simulink model "TSR_Scenario_005_cs"  (R2014b)
settings: Solver=ode5  SolverMode=SingleTasking  StartTime=0.0  StopTime=inf  FixedStep=1/100  RelTol=1e-3
PreLoadFcn:
  | mbxruntime.callbacks.PreLoadFcn(bdroot);
  | check_NUTS_defined;
  | 
  | assignin('base',['model_closed_' bdroot],false);
  | 
  | addpath('../includes_TSR/includes_TSR');
  | 
  | switch version('-release')
  | case {'2010a', '2010b', '2011a'}
  | addpath('../includes_TSR/ML2010b');
  | otherwise
  | addpath('../includes_TSR/ML2011b');
  | end
PostLoadFcn:
  | mbxruntime.callbacks.PostLoadFcn(bdroot);
InitFcn:
  | mbxruntime.callbacks.InitFcn(bdroot);
StartFcn:
  | mbxruntime.callbacks.StartFcn(bdroot);
StopFcn:
  | mbxruntime.callbacks.StopFcn(bdroot);
model workspace: external: MAT-File .\TSR_Scenario_005_cs_hws.mat (data not in the file)
undefined symbols (not defined in the file or in its folder): InitImageOutputDir, mbxruntime, OrientationPitch, OrientationRoll, PositionX, PositionY, PositionZ, tabledata, warningInitialVelocity, x0
undefined symbols (not defined in the file): SteeringColumn, SteeringWheel, TSR_Scenario_005_cs_00431f954bf6ed0a, TSR_Scenario_005_cs_02a6645fe307ce96, TSR_Scenario_005_cs_0e0d17e780cba748, TSR_Scenario_005_cs_0f94700004e304be, TSR_Scenario_005_cs_13e63084604f23c5, TSR_Scenario_005_cs_18da76569b226b1d, TSR_Scenario_005_cs_19a09eb0dceaf389, TSR_Scenario_005_cs_1d6b1ecf339da803, TSR_Scenario_005_cs_219485daa5a5d171, TSR_Scenario_005_cs_221c03cfb0670d1a, TSR_Scenario_005_cs_22611db63f83df91, TSR_Scenario_005_cs_24324341e1f0fdeb, TSR_Scenario_005_cs_248b5be6aaeb4a32, TSR_Scenario_005_cs_26d69342f02903e6, TSR_Scenario_005_cs_28d4639b4eb6a924, TSR_Scenario_005_cs_2a50646ef6121283, TSR_Scenario_005_cs_2addef8764f78195, TSR_Scenario_005_cs_2c78bb6e92f1c73d, TSR_Scenario_005_cs_330b013c7926b8c0, TSR_Scenario_005_cs_33ac55a3a4bfafc5, TSR_Scenario_005_cs_33d6442482a921b6, TSR_Scenario_005_cs_36fcc85960c1dc31, TSR_Scenario_005_cs_38acb22310967a91, TSR_Scenario_005_cs_3e8855054a9c05f5, TSR_Scenario_005_cs_43d01b44652f0f38, TSR_Scenario_005_cs_43d19ecb630bd754, TSR_Scenario_005_cs_4487c76a87b8c5f1, TSR_Scenario_005_cs_44ceee846c318dfb, TSR_Scenario_005_cs_450a3683cbfdd730, TSR_Scenario_005_cs_464618e49e37493a, TSR_Scenario_005_cs_4880b38df4698ab1, TSR_Scenario_005_cs_4a2b3c7d0abca22e, TSR_Scenario_005_cs_4bd204b8239d5406, TSR_Scenario_005_cs_4de8d67ffbf74a19, TSR_Scenario_005_cs_4f6170ee339e194e, TSR_Scenario_005_cs_50430c8166448bfc, TSR_Scenario_005_cs_53c8f6734eaacbd2, TSR_Scenario_005_cs_543db9a2ff458ebe, TSR_Scenario_005_cs_57976f30ab2edad5, TSR_Scenario_005_cs_5922fccf31372278, TSR_Scenario_005_cs_5a258c940bbe826b, TSR_Scenario_005_cs_6087cc283675db35, TSR_Scenario_005_cs_6246b869963d4acb, TSR_Scenario_005_cs_6352b9f9b72630f9, TSR_Scenario_005_cs_6559b64eceddc3ca, TSR_Scenario_005_cs_6832a8ea8fa66aa4, TSR_Scenario_005_cs_696d53dba69844e5, TSR_Scenario_005_cs_6cabbb37c4ac2dd1, TSR_Scenario_005_cs_6d528aa494c8a952, TSR_Scenario_005_cs_6d945b49f7234fd2, TSR_Scenario_005_cs_6e2ebc771acb2455, TSR_Scenario_005_cs_7897f864ad990cf0, TSR_Scenario_005_cs_7978c65fd141f076, TSR_Scenario_005_cs_7a9ba94120bbe2c7, TSR_Scenario_005_cs_7b108592703c2dc5, TSR_Scenario_005_cs_7cd2f5b09394b811, TSR_Scenario_005_cs_7e1904d085d8f37f, TSR_Scenario_005_cs_7e555208507e0618 ... (+95)
libraries: simulink_extras x59, PreScanSimulinkLibrary x43, simulink x29
(part 6 of 24)

== system TSR_Scenario_005_cs/Lightpost_27 ==
  note: Texture Resources for Light
      |
      | ID: resource name
      | 1: LightMap\HeadLight LB and HB.png: HeadLight LB and HB
      | 2: LightMap\HeadLight LB.png: HeadLight LB
      | 3: LightMap\GeneralLight.png: GeneralLight
      | 4: LightMap\BrakeLight.png: BrakeLight
      | 5: LightMap\RearLight.png: RearLight
      | 6: LightMap\HeadLight HB.png: HeadLight HB
  Light_Col : Constant  Tag=VisuLightConst  Value=[255 210 89]
  Light_ID : Constant  Tag=VisuLightConst  Value=[0]
  Light_Mux : Subsystem  Tag=mux/ActiveLight  mask(PreScan User Interface: VisuActiveLight){}
      mask help:
      | The VisuActiveLight block provides a way for detailed animation of Light Sources, such as the indicator, brake, fog and main lights of a vehicle, or a light post.
      |
      | For more information, please click Help.
      settings: DeleteFcn=PreScanBlockDeleteFcn;
      mask Help: eval('openHelp(209)')
  Light_Ori : Constant  Tag=VisuLightConst  Value=[0.000000 -0.000000 0.000000]
  Light_Pos : Constant  Tag=VisuLightConst  Value=[-0.038900 -0.000018 0.870000]
  Light_mscd : Constant  Tag=VisuLightConst  Value=[48.371371]
  Lightpost_27_Light : Outport  Tag=outport/Light  OutDataTypeStr=Bus: PRESCAN_VISULIGHTACTUATOR_DATA  SampleTime=1/100
  wires:
  Light_Mux/1(Lights) -> Lightpost_27_Light/1
  Light_mscd/1 -> Light_Mux/1(MSCD [Cd])
  Light_Pos/1 -> Light_Mux/2(Position (xyz) [m])
  Light_Ori/1 -> Light_Mux/3(Orientation (RPY) [deg])
  Light_Col/1 -> Light_Mux/4(Color [-])
  Light_ID/1 -> Light_Mux/5(TextureResourceID [-])

== system TSR_Scenario_005_cs/Lightpost_27_Light ==
  Lightpost_27_Light : Inport  Tag=inport/Light  OutDataTypeStr=Bus: PRESCAN_VISULIGHTACTUATOR_DATA  SampleTime=1/100  BusOutputAsStruct=on
  Actuator : S-Function  FunctionName=sfun_VisuLightActuator  Parameters=mbxruntime.parameters.convert(UniqueID), mbxruntime.parameters.convert(LightName), mbxruntime.parameters.convert(PivotName), mbxruntime.parameters.convert(TextureResources), mbxruntime.parameters.convert(ColorsObjectName), mbxruntime.parameters.convert(MeshOnColor), mbxruntime.parameters.convert(MeshOffColor),tabledata, TimeStep  EnableBusSupport=off  mask(PreScan Sink Block: VisuActiveLight){UniqueID=638, LightName=Lightpost_27.LightActuator_0_Light_ActiveLight, PivotName=Lightpost_27.Light, TextureResources={ '1' 'LightMap\HeadLight LB and HB.png' '2' 'LightMap\HeadLight LB.png' '3' 'LightMap\GeneralLight.png' '4' 'LightMap\BrakeLight.png' '5' 'LightMap\RearLight.png' '6' 'LightMap\HeadLight HB.png'}, ColorsObjectName=Lightpost_27.Light, MeshOnColor=[224  224  224  255  224  224  224  255  102  102  102  255  510  420  178  255], MeshOffColor=[224  224  224  255  224  224  224  255  102  102  102  255    0    0    0  255], TimeStep=1/100}
      mask prompts: UniqueID "Parent Unique Identifier"; LightName "Light"; PivotName "Pivot"; TextureResources "Texture Resources"; ColorsObjectName "Light Fixture Color Object"; MeshOnColor "Light Fixture On Color"; MeshOffColor "Light Fixture Off Color"; TimeStep "Simulink time step"
      mask help:
      | The VisuActiveLight block provides a way for detailed animation of Light Sources, such as the indicator, brake, fog and main lights of a vehicle, or a light post.
      |
      | For more information, please click Help.
      mask init:
      | [tabledata] = mbxruntime.parameters.table(UniqueID,LightName,PivotName,TextureResources,ColorsObjectName,MeshOnColor,MeshOffColor);
      mask Help: eval('openHelp(209)')
      mask Display: image(imread('HeadLight.png'))
  wires:
  Lightpost_27_Light/1 -> Actuator/1

== system TSR_Scenario_005_cs/Lightpost_2_Light ==
  Lightpost_2_Light : Inport  Tag=inport/Light  OutDataTypeStr=Bus: PRESCAN_VISULIGHTACTUATOR_DATA  SampleTime=1/100  BusOutputAsStruct=on
  Actuator : S-Function  FunctionName=sfun_VisuLightActuator  Parameters=mbxruntime.parameters.convert(UniqueID), mbxruntime.parameters.convert(LightName), mbxruntime.parameters.convert(PivotName), mbxruntime.parameters.convert(TextureResources), mbxruntime.parameters.convert(ColorsObjectName), mbxruntime.parameters.convert(MeshOnColor), mbxruntime.parameters.convert(MeshOffColor),tabledata, TimeStep  EnableBusSupport=off  mask(PreScan Sink Block: VisuActiveLight){UniqueID=148, LightName=Lightpost_2.LightActuator_0_Light_ActiveLight, PivotName=Lightpost_2.Light, TextureResources={ '1' 'LightMap\HeadLight LB and HB.png' '2' 'LightMap\HeadLight LB.png' '3' 'LightMap\GeneralLight.png' '4' 'LightMap\BrakeLight.png' '5' 'LightMap\RearLight.png' '6' 'LightMap\HeadLight HB.png'}, ColorsObjectName=Lightpost_2.Light, MeshOnColor=[224  224  224  255  224  224  224  255  102  102  102  255  510  420  178  255], MeshOffColor=[224  224  224  255  224  224  224  255  102  102  102  255    0    0    0  255], TimeStep=1/100}
      mask prompts: UniqueID "Parent Unique Identifier"; LightName "Light"; PivotName "Pivot"; TextureResources "Texture Resources"; ColorsObjectName "Light Fixture Color Object"; MeshOnColor "Light Fixture On Color"; MeshOffColor "Light Fixture Off Color"; TimeStep "Simulink time step"
      mask help:
      | The VisuActiveLight block provides a way for detailed animation of Light Sources, such as the indicator, brake, fog and main lights of a vehicle, or a light post.
      |
      | For more information, please click Help.
      mask init:
      | [tabledata] = mbxruntime.parameters.table(UniqueID,LightName,PivotName,TextureResources,ColorsObjectName,MeshOnColor,MeshOffColor);
      mask Help: eval('openHelp(209)')
      mask Display: image(imread('HeadLight.png'))
  wires:
  Lightpost_2_Light/1 -> Actuator/1

== system TSR_Scenario_005_cs/Lightpost_3 ==
  note: Texture Resources for Light
      |
      | ID: resource name
      | 1: LightMap\HeadLight LB and HB.png: HeadLight LB and HB
      | 2: LightMap\HeadLight LB.png: HeadLight LB
      | 3: LightMap\GeneralLight.png: GeneralLight
      | 4: LightMap\BrakeLight.png: BrakeLight
      | 5: LightMap\RearLight.png: RearLight
      | 6: LightMap\HeadLight HB.png: HeadLight HB
  Light_Col : Constant  Tag=VisuLightConst  Value=[255 210 89]
  Light_ID : Constant  Tag=VisuLightConst  Value=[0]
  Light_Mux : Subsystem  Tag=mux/ActiveLight  mask(PreScan User Interface: VisuActiveLight){}
      mask help:
      | The VisuActiveLight block provides a way for detailed animation of Light Sources, such as the indicator, brake, fog and main lights of a vehicle, or a light post.
      |
      | For more information, please click Help.
      settings: DeleteFcn=PreScanBlockDeleteFcn;
      mask Help: eval('openHelp(209)')
  Light_Ori : Constant  Tag=VisuLightConst  Value=[0.000000 -0.000000 0.000000]
  Light_Pos : Constant  Tag=VisuLightConst  Value=[-0.038900 -0.000018 0.870000]
  Light_mscd : Constant  Tag=VisuLightConst  Value=[48.371371]
  Lightpost_3_Light : Outport  Tag=outport/Light  OutDataTypeStr=Bus: PRESCAN_VISULIGHTACTUATOR_DATA  SampleTime=1/100
  wires:
  Light_Mux/1(Lights) -> Lightpost_3_Light/1
  Light_mscd/1 -> Light_Mux/1(MSCD [Cd])
  Light_Pos/1 -> Light_Mux/2(Position (xyz) [m])
  Light_Ori/1 -> Light_Mux/3(Orientation (RPY) [deg])
  Light_Col/1 -> Light_Mux/4(Color [-])
  Light_ID/1 -> Light_Mux/5(TextureResourceID [-])

== system TSR_Scenario_005_cs/Lightpost_34 ==
  note: Texture Resources for Light
      |
      | ID: resource name
      | 1: LightMap\HeadLight LB and HB.png: HeadLight LB and HB
      | 2: LightMap\HeadLight LB.png: HeadLight LB
      | 3: LightMap\GeneralLight.png: GeneralLight
      | 4: LightMap\BrakeLight.png: BrakeLight
      | 5: LightMap\RearLight.png: RearLight
      | 6: LightMap\HeadLight HB.png: HeadLight HB
  Light_Col : Constant  Tag=VisuLightConst  Value=[255 210 89]
  Light_ID : Constant  Tag=VisuLightConst  Value=[0]
  Light_Mux : Subsystem  Tag=mux/ActiveLight  mask(PreScan User Interface: VisuActiveLight){}
      mask help:
      | The VisuActiveLight block provides a way for detailed animation of Light Sources, such as the indicator, brake, fog and main lights of a vehicle, or a light post.
      |
      | For more information, please click Help.
      settings: DeleteFcn=PreScanBlockDeleteFcn;
      mask Help: eval('openHelp(209)')
  Light_Ori : Constant  Tag=VisuLightConst  Value=[0.000000 -0.000000 0.000000]
  Light_Pos : Constant  Tag=VisuLightConst  Value=[-0.038900 -0.000018 0.870000]
  Light_mscd : Constant  Tag=VisuLightConst  Value=[48.371371]
  Lightpost_34_Light : Outport  Tag=outport/Light  OutDataTypeStr=Bus: PRESCAN_VISULIGHTACTUATOR_DATA  SampleTime=1/100
  wires:
  Light_Mux/1(Lights) -> Lightpost_34_Light/1
  Light_mscd/1 -> Light_Mux/1(MSCD [Cd])
  Light_Pos/1 -> Light_Mux/2(Position (xyz) [m])
  Light_Ori/1 -> Light_Mux/3(Orientation (RPY) [deg])
  Light_Col/1 -> Light_Mux/4(Color [-])
  Light_ID/1 -> Light_Mux/5(TextureResourceID [-])

== system TSR_Scenario_005_cs/Lightpost_34_Light ==
  Lightpost_34_Light : Inport  Tag=inport/Light  OutDataTypeStr=Bus: PRESCAN_VISULIGHTACTUATOR_DATA  SampleTime=1/100  BusOutputAsStruct=on
  Actuator : S-Function  FunctionName=sfun_VisuLightActuator  Parameters=mbxruntime.parameters.convert(UniqueID), mbxruntime.parameters.convert(LightName), mbxruntime.parameters.convert(PivotName), mbxruntime.parameters.convert(TextureResources), mbxruntime.parameters.convert(ColorsObjectName), mbxruntime.parameters.convert(MeshOnColor), mbxruntime.parameters.convert(MeshOffColor),tabledata, TimeStep  EnableBusSupport=off  mask(PreScan Sink Block: VisuActiveLight){UniqueID=645, LightName=Lightpost_34.LightActuator_0_Light_ActiveLight, PivotName=Lightpost_34.Light, TextureResources={ '1' 'LightMap\HeadLight LB and HB.png' '2' 'LightMap\HeadLight LB.png' '3' 'LightMap\GeneralLight.png' '4' 'LightMap\BrakeLight.png' '5' 'LightMap\RearLight.png' '6' 'LightMap\HeadLight HB.png'}, ColorsObjectName=Lightpost_34.Light, MeshOnColor=[224  224  224  255  224  224  224  255  102  102  102  255  510  420  178  255], MeshOffColor=[224  224  224  255  224  224  224  255  102  102  102  255    0    0    0  255], TimeStep=1/100}
      mask prompts: UniqueID "Parent Unique Identifier"; LightName "Light"; PivotName "Pivot"; TextureResources "Texture Resources"; ColorsObjectName "Light Fixture Color Object"; MeshOnColor "Light Fixture On Color"; MeshOffColor "Light Fixture Off Color"; TimeStep "Simulink time step"
      mask help:
      | The VisuActiveLight block provides a way for detailed animation of Light Sources, such as the indicator, brake, fog and main lights of a vehicle, or a light post.
      |
      | For more information, please click Help.
      mask init:
      | [tabledata] = mbxruntime.parameters.table(UniqueID,LightName,PivotName,TextureResources,ColorsObjectName,MeshOnColor,MeshOffColor);
      mask Help: eval('openHelp(209)')
      mask Display: image(imread('HeadLight.png'))
  wires:
  Lightpost_34_Light/1 -> Actuator/1

== system TSR_Scenario_005_cs/Lightpost_36 ==
  note: Texture Resources for Light
      |
      | ID: resource name
      | 1: LightMap\HeadLight LB and HB.png: HeadLight LB and HB
      | 2: LightMap\HeadLight LB.png: HeadLight LB
      | 3: LightMap\GeneralLight.png: GeneralLight
      | 4: LightMap\BrakeLight.png: BrakeLight
      | 5: LightMap\RearLight.png: RearLight
      | 6: LightMap\HeadLight HB.png: HeadLight HB
  Light_Col : Constant  Tag=VisuLightConst  Value=[255 210 89]
  Light_ID : Constant  Tag=VisuLightConst  Value=[0]
  Light_Mux : Subsystem  Tag=mux/ActiveLight  mask(PreScan User Interface: VisuActiveLight){}
      mask help:
      | The VisuActiveLight block provides a way for detailed animation of Light Sources, such as the indicator, brake, fog and main lights of a vehicle, or a light post.
      |
      | For more information, please click Help.
      settings: DeleteFcn=PreScanBlockDeleteFcn;
      mask Help: eval('openHelp(209)')
  Light_Ori : Constant  Tag=VisuLightConst  Value=[0.000000 -0.000000 0.000000]
  Light_Pos : Constant  Tag=VisuLightConst  Value=[-0.038900 -0.000018 0.870000]
  Light_mscd : Constant  Tag=VisuLightConst  Value=[48.371371]
  Lightpost_36_Light : Outport  Tag=outport/Light  OutDataTypeStr=Bus: PRESCAN_VISULIGHTACTUATOR_DATA  SampleTime=1/100
  wires:
  Light_Mux/1(Lights) -> Lightpost_36_Light/1
  Light_mscd/1 -> Light_Mux/1(MSCD [Cd])
  Light_Pos/1 -> Light_Mux/2(Position (xyz) [m])
  Light_Ori/1 -> Light_Mux/3(Orientation (RPY) [deg])
  Light_Col/1 -> Light_Mux/4(Color [-])
  Light_ID/1 -> Light_Mux/5(TextureResourceID [-])

== system TSR_Scenario_005_cs/Lightpost_36_Light ==
  Lightpost_36_Light : Inport  Tag=inport/Light  OutDataTypeStr=Bus: PRESCAN_VISULIGHTACTUATOR_DATA  SampleTime=1/100  BusOutputAsStruct=on
  Actuator : S-Function  FunctionName=sfun_VisuLightActuator  Parameters=mbxruntime.parameters.convert(UniqueID), mbxruntime.parameters.convert(LightName), mbxruntime.parameters.convert(PivotName), mbxruntime.parameters.convert(TextureResources), mbxruntime.parameters.convert(ColorsObjectName), mbxruntime.parameters.convert(MeshOnColor), mbxruntime.parameters.convert(MeshOffColor),tabledata, TimeStep  EnableBusSupport=off  mask(PreScan Sink Block: VisuActiveLight){UniqueID=647, LightName=Lightpost_36.LightActuator_0_Light_ActiveLight, PivotName=Lightpost_36.Light, TextureResources={ '1' 'LightMap\HeadLight LB and HB.png' '2' 'LightMap\HeadLight LB.png' '3' 'LightMap\GeneralLight.png' '4' 'LightMap\BrakeLight.png' '5' 'LightMap\RearLight.png' '6' 'LightMap\HeadLight HB.png'}, ColorsObjectName=Lightpost_36.Light, MeshOnColor=[224  224  224  255  224  224  224  255  102  102  102  255  510  420  178  255], MeshOffColor=[224  224  224  255  224  224  224  255  102  102  102  255    0    0    0  255], TimeStep=1/100}
      mask prompts: UniqueID "Parent Unique Identifier"; LightName "Light"; PivotName "Pivot"; TextureResources "Texture Resources"; ColorsObjectName "Light Fixture Color Object"; MeshOnColor "Light Fixture On Color"; MeshOffColor "Light Fixture Off Color"; TimeStep "Simulink time step"
      mask help:
      | The VisuActiveLight block provides a way for detailed animation of Light Sources, such as the indicator, brake, fog and main lights of a vehicle, or a light post.
      |
      | For more information, please click Help.
      mask init:
      | [tabledata] = mbxruntime.parameters.table(UniqueID,LightName,PivotName,TextureResources,ColorsObjectName,MeshOnColor,MeshOffColor);
      mask Help: eval('openHelp(209)')
      mask Display: image(imread('HeadLight.png'))
  wires:
  Lightpost_36_Light/1 -> Actuator/1

== system TSR_Scenario_005_cs/Lightpost_38 ==
  note: Texture Resources for Light
      |
      | ID: resource name
      | 1: LightMap\HeadLight LB and HB.png: HeadLight LB and HB
      | 2: LightMap\HeadLight LB.png: HeadLight LB
      | 3: LightMap\GeneralLight.png: GeneralLight
      | 4: LightMap\BrakeLight.png: BrakeLight
      | 5: LightMap\RearLight.png: RearLight
      | 6: LightMap\HeadLight HB.png: HeadLight HB
  Light_Col : Constant  Tag=VisuLightConst  Value=[255 210 89]
  Light_ID : Constant  Tag=VisuLightConst  Value=[0]
  Light_Mux : Subsystem  Tag=mux/ActiveLight  mask(PreScan User Interface: VisuActiveLight){}
      mask help:
      | The VisuActiveLight block provides a way for detailed animation of Light Sources, such as the indicator, brake, fog and main lights of a vehicle, or a light post.
      |
      | For more information, please click Help.
      settings: DeleteFcn=PreScanBlockDeleteFcn;
      mask Help: eval('openHelp(209)')
  Light_Ori : Constant  Tag=VisuLightConst  Value=[0.000000 -0.000000 0.000000]
  Light_Pos : Constant  Tag=VisuLightConst  Value=[-0.038900 -0.000018 0.870000]
  Light_mscd : Constant  Tag=VisuLightConst  Value=[48.371371]
  Lightpost_38_Light : Outport  Tag=outport/Light  OutDataTypeStr=Bus: PRESCAN_VISULIGHTACTUATOR_DATA  SampleTime=1/100
  wires:
  Light_Mux/1(Lights) -> Lightpost_38_Light/1
  Light_mscd/1 -> Light_Mux/1(MSCD [Cd])
  Light_Pos/1 -> Light_Mux/2(Position (xyz) [m])
  Light_Ori/1 -> Light_Mux/3(Orientation (RPY) [deg])
  Light_Col/1 -> Light_Mux/4(Color [-])
  Light_ID/1 -> Light_Mux/5(TextureResourceID [-])

== system TSR_Scenario_005_cs/Lightpost_38_Light ==
  Lightpost_38_Light : Inport  Tag=inport/Light  OutDataTypeStr=Bus: PRESCAN_VISULIGHTACTUATOR_DATA  SampleTime=1/100  BusOutputAsStruct=on
  Actuator : S-Function  FunctionName=sfun_VisuLightActuator  Parameters=mbxruntime.parameters.convert(UniqueID), mbxruntime.parameters.convert(LightName), mbxruntime.parameters.convert(PivotName), mbxruntime.parameters.convert(TextureResources), mbxruntime.parameters.convert(ColorsObjectName), mbxruntime.parameters.convert(MeshOnColor), mbxruntime.parameters.convert(MeshOffColor),tabledata, TimeStep  EnableBusSupport=off  mask(PreScan Sink Block: VisuActiveLight){UniqueID=649, LightName=Lightpost_38.LightActuator_0_Light_ActiveLight, PivotName=Lightpost_38.Light, TextureResources={ '1' 'LightMap\HeadLight LB and HB.png' '2' 'LightMap\HeadLight LB.png' '3' 'LightMap\GeneralLight.png' '4' 'LightMap\BrakeLight.png' '5' 'LightMap\RearLight.png' '6' 'LightMap\HeadLight HB.png'}, ColorsObjectName=Lightpost_38.Light, MeshOnColor=[224  224  224  255  224  224  224  255  102  102  102  255  510  420  178  255], MeshOffColor=[224  224  224  255  224  224  224  255  102  102  102  255    0    0    0  255], TimeStep=1/100}
      mask prompts: UniqueID "Parent Unique Identifier"; LightName "Light"; PivotName "Pivot"; TextureResources "Texture Resources"; ColorsObjectName "Light Fixture Color Object"; MeshOnColor "Light Fixture On Color"; MeshOffColor "Light Fixture Off Color"; TimeStep "Simulink time step"
      mask help:
      | The VisuActiveLight block provides a way for detailed animation of Light Sources, such as the indicator, brake, fog and main lights of a vehicle, or a light post.
      |
      | For more information, please click Help.
      mask init:
      | [tabledata] = mbxruntime.parameters.table(UniqueID,LightName,PivotName,TextureResources,ColorsObjectName,MeshOnColor,MeshOffColor);
      mask Help: eval('openHelp(209)')
      mask Display: image(imread('HeadLight.png'))
  wires:
  Lightpost_38_Light/1 -> Actuator/1

== system TSR_Scenario_005_cs/Lightpost_3_Light ==
  Lightpost_3_Light : Inport  Tag=inport/Light  OutDataTypeStr=Bus: PRESCAN_VISULIGHTACTUATOR_DATA  SampleTime=1/100  BusOutputAsStruct=on
  Actuator : S-Function  FunctionName=sfun_VisuLightActuator  Parameters=mbxruntime.parameters.convert(UniqueID), mbxruntime.parameters.convert(LightName), mbxruntime.parameters.convert(PivotName), mbxruntime.parameters.convert(TextureResources), mbxruntime.parameters.convert(ColorsObjectName), mbxruntime.parameters.convert(MeshOnColor), mbxruntime.parameters.convert(MeshOffColor),tabledata, TimeStep  EnableBusSupport=off  mask(PreScan Sink Block: VisuActiveLight){UniqueID=150, LightName=Lightpost_3.LightActuator_0_Light_ActiveLight, PivotName=Lightpost_3.Light, TextureResources={ '1' 'LightMap\HeadLight LB and HB.png' '2' 'LightMap\HeadLight LB.png' '3' 'LightMap\GeneralLight.png' '4' 'LightMap\BrakeLight.png' '5' 'LightMap\RearLight.png' '6' 'LightMap\HeadLight HB.png'}, ColorsObjectName=Lightpost_3.Light, MeshOnColor=[224  224  224  255  224  224  224  255  102  102  102  255  510  420  178  255], MeshOffColor=[224  224  224  255  224  224  224  255  102  102  102  255    0    0    0  255], TimeStep=1/100}
      mask prompts: UniqueID "Parent Unique Identifier"; LightName "Light"; PivotName "Pivot"; TextureResources "Texture Resources"; ColorsObjectName "Light Fixture Color Object"; MeshOnColor "Light Fixture On Color"; MeshOffColor "Light Fixture Off Color"; TimeStep "Simulink time step"
      mask help:
      | The VisuActiveLight block provides a way for detailed animation of Light Sources, such as the indicator, brake, fog and main lights of a vehicle, or a light post.
      |
      | For more information, please click Help.
      mask init:
      | [tabledata] = mbxruntime.parameters.table(UniqueID,LightName,PivotName,TextureResources,ColorsObjectName,MeshOnColor,MeshOffColor);
      mask Help: eval('openHelp(209)')
      mask Display: image(imread('HeadLight.png'))
  wires:
  Lightpost_3_Light/1 -> Actuator/1

== system TSR_Scenario_005_cs/Lightpost_4 ==
  note: Texture Resources for Light
      |
      | ID: resource name
      | 1: LightMap\HeadLight LB and HB.png: HeadLight LB and HB
      | 2: LightMap\HeadLight LB.png: HeadLight LB
      | 3: LightMap\GeneralLight.png: GeneralLight
      | 4: LightMap\BrakeLight.png: BrakeLight
      | 5: LightMap\RearLight.png: RearLight
      | 6: LightMap\HeadLight HB.png: HeadLight HB
  Light_Col : Constant  Tag=VisuLightConst  Value=[255 210 89]
  Light_ID : Constant  Tag=VisuLightConst  Value=[0]
  Light_Mux : Subsystem  Tag=mux/ActiveLight  mask(PreScan User Interface: VisuActiveLight){}
      mask help:
      | The VisuActiveLight block provides a way for detailed animation of Light Sources, such as the indicator, brake, fog and main lights of a vehicle, or a light post.
      |
      | For more information, please click Help.
      settings: DeleteFcn=PreScanBlockDeleteFcn;
      mask Help: eval('openHelp(209)')
  Light_Ori : Constant  Tag=VisuLightConst  Value=[0.000000 -0.000000 0.000000]
  Light_Pos : Constant  Tag=VisuLightConst  Value=[-0.038900 -0.000018 0.870000]
  Light_mscd : Constant  Tag=VisuLightConst  Value=[48.371371]
  Lightpost_4_Light : Outport  Tag=outport/Light  OutDataTypeStr=Bus: PRESCAN_VISULIGHTACTUATOR_DATA  SampleTime=1/100
  wires:
  Light_Mux/1(Lights) -> Lightpost_4_Light/1
  Light_mscd/1 -> Light_Mux/1(MSCD [Cd])
  Light_Pos/1 -> Light_Mux/2(Position (xyz) [m])
  Light_Ori/1 -> Light_Mux/3(Orientation (RPY) [deg])
  Light_Col/1 -> Light_Mux/4(Color [-])
  Light_ID/1 -> Light_Mux/5(TextureResourceID [-])

== system TSR_Scenario_005_cs/Lightpost_40 ==
  note: Texture Resources for Light
      |
      | ID: resource name
      | 1: LightMap\HeadLight LB and HB.png: HeadLight LB and HB
      | 2: LightMap\HeadLight LB.png: HeadLight LB
      | 3: LightMap\GeneralLight.png: GeneralLight
      | 4: LightMap\BrakeLight.png: BrakeLight
      | 5: LightMap\RearLight.png: RearLight
      | 6: LightMap\HeadLight HB.png: HeadLight HB
  Light_Col : Constant  Tag=VisuLightConst  Value=[255 210 89]
  Light_ID : Constant  Tag=VisuLightConst  Value=[0]
  Light_Mux : Subsystem  Tag=mux/ActiveLight  mask(PreScan User Interface: VisuActiveLight){}
      mask help:
      | The VisuActiveLight block provides a way for detailed animation of Light Sources, such as the indicator, brake, fog and main lights of a vehicle, or a light post.
      |
      | For more information, please click Help.
      settings: DeleteFcn=PreScanBlockDeleteFcn;
      mask Help: eval('openHelp(209)')
  Light_Ori : Constant  Tag=VisuLightConst  Value=[0.000000 -0.000000 0.000000]
  Light_Pos : Constant  Tag=VisuLightConst  Value=[-0.038900 -0.000018 0.870000]
  Light_mscd : Constant  Tag=VisuLightConst  Value=[48.371371]
  Lightpost_40_Light : Outport  Tag=outport/Light  OutDataTypeStr=Bus: PRESCAN_VISULIGHTACTUATOR_DATA  SampleTime=1/100
  wires:
  Light_Mux/1(Lights) -> Lightpost_40_Light/1
  Light_mscd/1 -> Light_Mux/1(MSCD [Cd])
  Light_Pos/1 -> Light_Mux/2(Position (xyz) [m])
  Light_Ori/1 -> Light_Mux/3(Orientation (RPY) [deg])
  Light_Col/1 -> Light_Mux/4(Color [-])
  Light_ID/1 -> Light_Mux/5(TextureResourceID [-])

== system TSR_Scenario_005_cs/Lightpost_40_Light ==
  Lightpost_40_Light : Inport  Tag=inport/Light  OutDataTypeStr=Bus: PRESCAN_VISULIGHTACTUATOR_DATA  SampleTime=1/100  BusOutputAsStruct=on
  Actuator : S-Function  FunctionName=sfun_VisuLightActuator  Parameters=mbxruntime.parameters.convert(UniqueID), mbxruntime.parameters.convert(LightName), mbxruntime.parameters.convert(PivotName), mbxruntime.parameters.convert(TextureResources), mbxruntime.parameters.convert(ColorsObjectName), mbxruntime.parameters.convert(MeshOnColor), mbxruntime.parameters.convert(MeshOffColor),tabledata, TimeStep  EnableBusSupport=off  mask(PreScan Sink Block: VisuActiveLight){UniqueID=651, LightName=Lightpost_40.LightActuator_0_Light_ActiveLight, PivotName=Lightpost_40.Light, TextureResources={ '1' 'LightMap\HeadLight LB and HB.png' '2' 'LightMap\HeadLight LB.png' '3' 'LightMap\GeneralLight.png' '4' 'LightMap\BrakeLight.png' '5' 'LightMap\RearLight.png' '6' 'LightMap\HeadLight HB.png'}, ColorsObjectName=Lightpost_40.Light, MeshOnColor=[224  224  224  255  224  224  224  255  102  102  102  255  510  420  178  255], MeshOffColor=[224  224  224  255  224  224  224  255  102  102  102  255    0    0    0  255], TimeStep=1/100}
      mask prompts: UniqueID "Parent Unique Identifier"; LightName "Light"; PivotName "Pivot"; TextureResources "Texture Resources"; ColorsObjectName "Light Fixture Color Object"; MeshOnColor "Light Fixture On Color"; MeshOffColor "Light Fixture Off Color"; TimeStep "Simulink time step"
      mask help:
      | The VisuActiveLight block provides a way for detailed animation of Light Sources, such as the indicator, brake, fog and main lights of a vehicle, or a light post.
      |
      | For more information, please click Help.
      mask init:
      | [tabledata] = mbxruntime.parameters.table(UniqueID,LightName,PivotName,TextureResources,ColorsObjectName,MeshOnColor,MeshOffColor);
      mask Help: eval('openHelp(209)')
      mask Display: image(imread('HeadLight.png'))
  wires:
  Lightpost_40_Light/1 -> Actuator/1

== system TSR_Scenario_005_cs/Lightpost_42 ==
  note: Texture Resources for Light
      |
      | ID: resource name
      | 1: LightMap\HeadLight LB and HB.png: HeadLight LB and HB
      | 2: LightMap\HeadLight LB.png: HeadLight LB
      | 3: LightMap\GeneralLight.png: GeneralLight
      | 4: LightMap\BrakeLight.png: BrakeLight
      | 5: LightMap\RearLight.png: RearLight
      | 6: LightMap\HeadLight HB.png: HeadLight HB
  Light_Col : Constant  Tag=VisuLightConst  Value=[255 210 89]
  Light_ID : Constant  Tag=VisuLightConst  Value=[0]
  Light_Mux : Subsystem  Tag=mux/ActiveLight  mask(PreScan User Interface: VisuActiveLight){}
      mask help:
      | The VisuActiveLight block provides a way for detailed animation of Light Sources, such as the indicator, brake, fog and main lights of a vehicle, or a light post.
      |
      | For more information, please click Help.
      settings: DeleteFcn=PreScanBlockDeleteFcn;
      mask Help: eval('openHelp(209)')
  Light_Ori : Constant  Tag=VisuLightConst  Value=[0.000000 -0.000000 0.000000]
  Light_Pos : Constant  Tag=VisuLightConst  Value=[-0.038900 -0.000018 0.870000]
  Light_mscd : Constant  Tag=VisuLightConst  Value=[48.371371]
  Lightpost_42_Light : Outport  Tag=outport/Light  OutDataTypeStr=Bus: PRESCAN_VISULIGHTACTUATOR_DATA  SampleTime=1/100
  wires:
  Light_Mux/1(Lights) -> Lightpost_42_Light/1
  Light_mscd/1 -> Light_Mux/1(MSCD [Cd])
  Light_Pos/1 -> Light_Mux/2(Position (xyz) [m])
  Light_Ori/1 -> Light_Mux/3(Orientation (RPY) [deg])
  Light_Col/1 -> Light_Mux/4(Color [-])
  Light_ID/1 -> Light_Mux/5(TextureResourceID [-])

== system TSR_Scenario_005_cs/Lightpost_42_Light ==
  Lightpost_42_Light : Inport  Tag=inport/Light  OutDataTypeStr=Bus: PRESCAN_VISULIGHTACTUATOR_DATA  SampleTime=1/100  BusOutputAsStruct=on
  Actuator : S-Function  FunctionName=sfun_VisuLightActuator  Parameters=mbxruntime.parameters.convert(UniqueID), mbxruntime.parameters.convert(LightName), mbxruntime.parameters.convert(PivotName), mbxruntime.parameters.convert(TextureResources), mbxruntime.parameters.convert(ColorsObjectName), mbxruntime.parameters.convert(MeshOnColor), mbxruntime.parameters.convert(MeshOffColor),tabledata, TimeStep  EnableBusSupport=off  mask(PreScan Sink Block: VisuActiveLight){UniqueID=653, LightName=Lightpost_42.LightActuator_0_Light_ActiveLight, PivotName=Lightpost_42.Light, TextureResources={ '1' 'LightMap\HeadLight LB and HB.png' '2' 'LightMap\HeadLight LB.png' '3' 'LightMap\GeneralLight.png' '4' 'LightMap\BrakeLight.png' '5' 'LightMap\RearLight.png' '6' 'LightMap\HeadLight HB.png'}, ColorsObjectName=Lightpost_42.Light, MeshOnColor=[224  224  224  255  224  224  224  255  102  102  102  255  510  420  178  255], MeshOffColor=[224  224  224  255  224  224  224  255  102  102  102  255    0    0    0  255], TimeStep=1/100}
      mask prompts: UniqueID "Parent Unique Identifier"; LightName "Light"; PivotName "Pivot"; TextureResources "Texture Resources"; ColorsObjectName "Light Fixture Color Object"; MeshOnColor "Light Fixture On Color"; MeshOffColor "Light Fixture Off Color"; TimeStep "Simulink time step"
      mask help:
      | The VisuActiveLight block provides a way for detailed animation of Light Sources, such as the indicator, brake, fog and main lights of a vehicle, or a light post.
      |
      | For more information, please click Help.
      mask init:
      | [tabledata] = mbxruntime.parameters.table(UniqueID,LightName,PivotName,TextureResources,ColorsObjectName,MeshOnColor,MeshOffColor);
      mask Help: eval('openHelp(209)')
      mask Display: image(imread('HeadLight.png'))
  wires:
  Lightpost_42_Light/1 -> Actuator/1

== system TSR_Scenario_005_cs/Lightpost_44 ==
  note: Texture Resources for Light
      |
      | ID: resource name
      | 1: LightMap\HeadLight LB and HB.png: HeadLight LB and HB
      | 2: LightMap\HeadLight LB.png: HeadLight LB
      | 3: LightMap\GeneralLight.png: GeneralLight
      | 4: LightMap\BrakeLight.png: BrakeLight
      | 5: LightMap\RearLight.png: RearLight
      | 6: LightMap\HeadLight HB.png: HeadLight HB
  Light_Col : Constant  Tag=VisuLightConst  Value=[255 210 89]
  Light_ID : Constant  Tag=VisuLightConst  Value=[0]
  Light_Mux : Subsystem  Tag=mux/ActiveLight  mask(PreScan User Interface: VisuActiveLight){}
      mask help:
      | The VisuActiveLight block provides a way for detailed animation of Light Sources, such as the indicator, brake, fog and main lights of a vehicle, or a light post.
      |
      | For more information, please click Help.
      settings: DeleteFcn=PreScanBlockDeleteFcn;
      mask Help: eval('openHelp(209)')
  Light_Ori : Constant  Tag=VisuLightConst  Value=[0.000000 -0.000000 0.000000]
  Light_Pos : Constant  Tag=VisuLightConst  Value=[-0.038900 -0.000018 0.870000]
  Light_mscd : Constant  Tag=VisuLightConst  Value=[48.371371]
  Lightpost_44_Light : Outport  Tag=outport/Light  OutDataTypeStr=Bus: PRESCAN_VISULIGHTACTUATOR_DATA  SampleTime=1/100
  wires:
  Light_Mux/1(Lights) -> Lightpost_44_Light/1
  Light_mscd/1 -> Light_Mux/1(MSCD [Cd])
  Light_Pos/1 -> Light_Mux/2(Position (xyz) [m])
  Light_Ori/1 -> Light_Mux/3(Orientation (RPY) [deg])
  Light_Col/1 -> Light_Mux/4(Color [-])
  Light_ID/1 -> Light_Mux/5(TextureResourceID [-])

== system TSR_Scenario_005_cs/Lightpost_44_Light ==
  Lightpost_44_Light : Inport  Tag=inport/Light  OutDataTypeStr=Bus: PRESCAN_VISULIGHTACTUATOR_DATA  SampleTime=1/100  BusOutputAsStruct=on
  Actuator : S-Function  FunctionName=sfun_VisuLightActuator  Parameters=mbxruntime.parameters.convert(UniqueID), mbxruntime.parameters.convert(LightName), mbxruntime.parameters.convert(PivotName), mbxruntime.parameters.convert(TextureResources), mbxruntime.parameters.convert(ColorsObjectName), mbxruntime.parameters.convert(MeshOnColor), mbxruntime.parameters.convert(MeshOffColor),tabledata, TimeStep  EnableBusSupport=off  mask(PreScan Sink Block: VisuActiveLight){UniqueID=655, LightName=Lightpost_44.LightActuator_0_Light_ActiveLight, PivotName=Lightpost_44.Light, TextureResources={ '1' 'LightMap\HeadLight LB and HB.png' '2' 'LightMap\HeadLight LB.png' '3' 'LightMap\GeneralLight.png' '4' 'LightMap\BrakeLight.png' '5' 'LightMap\RearLight.png' '6' 'LightMap\HeadLight HB.png'}, ColorsObjectName=Lightpost_44.Light, MeshOnColor=[224  224  224  255  224  224  224  255  102  102  102  255  510  420  178  255], MeshOffColor=[224  224  224  255  224  224  224  255  102  102  102  255    0    0    0  255], TimeStep=1/100}
      mask prompts: UniqueID "Parent Unique Identifier"; LightName "Light"; PivotName "Pivot"; TextureResources "Texture Resources"; ColorsObjectName "Light Fixture Color Object"; MeshOnColor "Light Fixture On Color"; MeshOffColor "Light Fixture Off Color"; TimeStep "Simulink time step"
      mask help:
      | The VisuActiveLight block provides a way for detailed animation of Light Sources, such as the indicator, brake, fog and main lights of a vehicle, or a light post.
      |
      | For more information, please click Help.
      mask init:
      | [tabledata] = mbxruntime.parameters.table(UniqueID,LightName,PivotName,TextureResources,ColorsObjectName,MeshOnColor,MeshOffColor);
      mask Help: eval('openHelp(209)')
      mask Display: image(imread('HeadLight.png'))
  wires:
  Lightpost_44_Light/1 -> Actuator/1

== system TSR_Scenario_005_cs/Lightpost_4_Light ==
  Lightpost_4_Light : Inport  Tag=inport/Light  OutDataTypeStr=Bus: PRESCAN_VISULIGHTACTUATOR_DATA  SampleTime=1/100  BusOutputAsStruct=on
  Actuator : S-Function  FunctionName=sfun_VisuLightActuator  Parameters=mbxruntime.parameters.convert(UniqueID), mbxruntime.parameters.convert(LightName), mbxruntime.parameters.convert(PivotName), mbxruntime.parameters.convert(TextureResources), mbxruntime.parameters.convert(ColorsObjectName), mbxruntime.parameters.convert(MeshOnColor), mbxruntime.parameters.convert(MeshOffColor),tabledata, TimeStep  EnableBusSupport=off  mask(PreScan Sink Block: VisuActiveLight){UniqueID=151, LightName=Lightpost_4.LightActuator_0_Light_ActiveLight, PivotName=Lightpost_4.Light, TextureResources={ '1' 'LightMap\HeadLight LB and HB.png' '2' 'LightMap\HeadLight LB.png' '3' 'LightMap\GeneralLight.png' '4' 'LightMap\BrakeLight.png' '5' 'LightMap\RearLight.png' '6' 'LightMap\HeadLight HB.png'}, ColorsObjectName=Lightpost_4.Light, MeshOnColor=[224  224  224  255  224  224  224  255  102  102  102  255  510  420  178  255], MeshOffColor=[224  224  224  255  224  224  224  255  102  102  102  255    0    0    0  255], TimeStep=1/100}
      mask prompts: UniqueID "Parent Unique Identifier"; LightName "Light"; PivotName "Pivot"; TextureResources "Texture Resources"; ColorsObjectName "Light Fixture Color Object"; MeshOnColor "Light Fixture On Color"; MeshOffColor "Light Fixture Off Color"; TimeStep "Simulink time step"
      mask help:
      | The VisuActiveLight block provides a way for detailed animation of Light Sources, such as the indicator, brake, fog and main lights of a vehicle, or a light post.
      |
      | For more information, please click Help.
      mask init:
      | [tabledata] = mbxruntime.parameters.table(UniqueID,LightName,PivotName,TextureResources,ColorsObjectName,MeshOnColor,MeshOffColor);
      mask Help: eval('openHelp(209)')
      mask Display: image(imread('HeadLight.png'))
  wires:
  Lightpost_4_Light/1 -> Actuator/1

== system TSR_Scenario_005_cs/Lightpost_5 ==
  note: Texture Resources for Light
      |
      | ID: resource name
      | 1: LightMap\HeadLight LB and HB.png: HeadLight LB and HB
      | 2: LightMap\HeadLight LB.png: HeadLight LB
      | 3: LightMap\GeneralLight.png: GeneralLight
      | 4: LightMap\BrakeLight.png: BrakeLight
      | 5: LightMap\RearLight.png: RearLight
      | 6: LightMap\HeadLight HB.png: HeadLight HB
  Light_Col : Constant  Tag=VisuLightConst  Value=[255 210 89]
  Light_ID : Constant  Tag=VisuLightConst  Value=[0]
  Light_Mux : Subsystem  Tag=mux/ActiveLight  mask(PreScan User Interface: VisuActiveLight){}
      mask help:
      | The VisuActiveLight block provides a way for detailed animation of Light Sources, such as the indicator, brake, fog and main lights of a vehicle, or a light post.
      |
      | For more information, please click Help.
      settings: DeleteFcn=PreScanBlockDeleteFcn;
      mask Help: eval('openHelp(209)')
  Light_Ori : Constant  Tag=VisuLightConst  Value=[0.000000 -0.000000 0.000000]
  Light_Pos : Constant  Tag=VisuLightConst  Value=[-0.038900 -0.000018 0.870000]
  Light_mscd : Constant  Tag=VisuLightConst  Value=[48.371371]
  Lightpost_5_Light : Outport  Tag=outport/Light  OutDataTypeStr=Bus: PRESCAN_VISULIGHTACTUATOR_DATA  SampleTime=1/100
  wires:
  Light_Mux/1(Lights) -> Lightpost_5_Light/1
  Light_mscd/1 -> Light_Mux/1(MSCD [Cd])
  Light_Pos/1 -> Light_Mux/2(Position (xyz) [m])
  Light_Ori/1 -> Light_Mux/3(Orientation (RPY) [deg])
  Light_Col/1 -> Light_Mux/4(Color [-])
  Light_ID/1 -> Light_Mux/5(TextureResourceID [-])

== system TSR_Scenario_005_cs/Lightpost_54 ==
  note: Texture Resources for Light
      |
      | ID: resource name
      | 1: LightMap\HeadLight LB and HB.png: HeadLight LB and HB
      | 2: LightMap\HeadLight LB.png: HeadLight LB
      | 3: LightMap\GeneralLight.png: GeneralLight
      | 4: LightMap\BrakeLight.png: BrakeLight
      | 5: LightMap\RearLight.png: RearLight
      | 6: LightMap\HeadLight HB.png: HeadLight HB
  Light_Col : Constant  Tag=VisuLightConst  Value=[255 210 89]
  Light_ID : Constant  Tag=VisuLightConst  Value=[0]
  Light_Mux : Subsystem  Tag=mux/ActiveLight  mask(PreScan User Interface: VisuActiveLight){}
      mask help:
      | The VisuActiveLight block provides a way for detailed animation of Light Sources, such as the indicator, brake, fog and main lights of a vehicle, or a light post.
      |
      | For more information, please click Help.
      settings: DeleteFcn=PreScanBlockDeleteFcn;
      mask Help: eval('openHelp(209)')
  Light_Ori : Constant  Tag=VisuLightConst  Value=[0.000000 -0.000000 0.000000]
  Light_Pos : Constant  Tag=VisuLightConst  Value=[-0.038900 -0.000018 0.870000]
  Light_mscd : Constant  Tag=VisuLightConst  Value=[48.371371]
  Lightpost_54_Light : Outport  Tag=outport/Light  OutDataTypeStr=Bus: PRESCAN_VISULIGHTACTUATOR_DATA  SampleTime=1/100
  wires:
  Light_Mux/1(Lights) -> Lightpost_54_Light/1
  Light_mscd/1 -> Light_Mux/1(MSCD [Cd])
  Light_Pos/1 -> Light_Mux/2(Position (xyz) [m])
  Light_Ori/1 -> Light_Mux/3(Orientation (RPY) [deg])
  Light_Col/1 -> Light_Mux/4(Color [-])
  Light_ID/1 -> Light_Mux/5(TextureResourceID [-])

== system TSR_Scenario_005_cs/Lightpost_54_Light ==
  Lightpost_54_Light : Inport  Tag=inport/Light  OutDataTypeStr=Bus: PRESCAN_VISULIGHTACTUATOR_DATA  SampleTime=1/100  BusOutputAsStruct=on
  Actuator : S-Function  FunctionName=sfun_VisuLightActuator  Parameters=mbxruntime.parameters.convert(UniqueID), mbxruntime.parameters.convert(LightName), mbxruntime.parameters.convert(PivotName), mbxruntime.parameters.convert(TextureResources), mbxruntime.parameters.convert(ColorsObjectName), mbxruntime.parameters.convert(MeshOnColor), mbxruntime.parameters.convert(MeshOffColor),tabledata, TimeStep  EnableBusSupport=off  mask(PreScan Sink Block: VisuActiveLight){UniqueID=712, LightName=Lightpost_54.LightActuator_0_Light_ActiveLight, PivotName=Lightpost_54.Light, TextureResources={ '1' 'LightMap\HeadLight LB and HB.png' '2' 'LightMap\HeadLight LB.png' '3' 'LightMap\GeneralLight.png' '4' 'LightMap\BrakeLight.png' '5' 'LightMap\RearLight.png' '6' 'LightMap\HeadLight HB.png'}, ColorsObjectName=Lightpost_54.Light, MeshOnColor=[224  224  224  255  224  224  224  255  102  102  102  255  510  420  178  255], MeshOffColor=[224  224  224  255  224  224  224  255  102  102  102  255    0    0    0  255], TimeStep=1/100}
      mask prompts: UniqueID "Parent Unique Identifier"; LightName "Light"; PivotName "Pivot"; TextureResources "Texture Resources"; ColorsObjectName "Light Fixture Color Object"; MeshOnColor "Light Fixture On Color"; MeshOffColor "Light Fixture Off Color"; TimeStep "Simulink time step"
      mask help:
      | The VisuActiveLight block provides a way for detailed animation of Light Sources, such as the indicator, brake, fog and main lights of a vehicle, or a light post.
      |
      | For more information, please click Help.
      mask init:
      | [tabledata] = mbxruntime.parameters.table(UniqueID,LightName,PivotName,TextureResources,ColorsObjectName,MeshOnColor,MeshOffColor);
      mask Help: eval('openHelp(209)')
      mask Display: image(imread('HeadLight.png'))
  wires:
  Lightpost_54_Light/1 -> Actuator/1

== system TSR_Scenario_005_cs/Lightpost_5_Light ==
  Lightpost_5_Light : Inport  Tag=inport/Light  OutDataTypeStr=Bus: PRESCAN_VISULIGHTACTUATOR_DATA  SampleTime=1/100  BusOutputAsStruct=on
  Actuator : S-Function  FunctionName=sfun_VisuLightActuator  Parameters=mbxruntime.parameters.convert(UniqueID), mbxruntime.parameters.convert(LightName), mbxruntime.parameters.convert(PivotName), mbxruntime.parameters.convert(TextureResources), mbxruntime.parameters.convert(ColorsObjectName), mbxruntime.parameters.convert(MeshOnColor), mbxruntime.parameters.convert(MeshOffColor),tabledata, TimeStep  EnableBusSupport=off  mask(PreScan Sink Block: VisuActiveLight){UniqueID=152, LightName=Lightpost_5.LightActuator_0_Light_ActiveLight, PivotName=Lightpost_5.Light, TextureResources={ '1' 'LightMap\HeadLight LB and HB.png' '2' 'LightMap\HeadLight LB.png' '3' 'LightMap\GeneralLight.png' '4' 'LightMap\BrakeLight.png' '5' 'LightMap\RearLight.png' '6' 'LightMap\HeadLight HB.png'}, ColorsObjectName=Lightpost_5.Light, MeshOnColor=[224  224  224  255  224  224  224  255  102  102  102  255  510  420  178  255], MeshOffColor=[224  224  224  255  224  224  224  255  102  102  102  255    0    0    0  255], TimeStep=1/100}
      mask prompts: UniqueID "Parent Unique Identifier"; LightName "Light"; PivotName "Pivot"; TextureResources "Texture Resources"; ColorsObjectName "Light Fixture Color Object"; MeshOnColor "Light Fixture On Color"; MeshOffColor "Light Fixture Off Color"; TimeStep "Simulink time step"
      mask help:
      | The VisuActiveLight block provides a way for detailed animation of Light Sources, such as the indicator, brake, fog and main lights of a vehicle, or a light post.
      |
      | For more information, please click Help.
      mask init:
      | [tabledata] = mbxruntime.parameters.table(UniqueID,LightName,PivotName,TextureResources,ColorsObjectName,MeshOnColor,MeshOffColor);
      mask Help: eval('openHelp(209)')
      mask Display: image(imread('HeadLight.png'))
  wires:
  Lightpost_5_Light/1 -> Actuator/1
